simulink model "VendingMachine"  (R2025a)
settings: Solver=VariableStepAuto  StartTime=0.0  StopTime=Inf  RelTol=1e-3
settings Model: Creator=Soochan Kim  LastModifiedBy=Soochan Kim

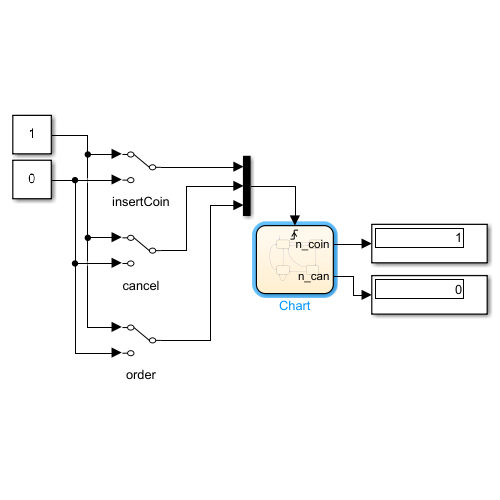
[thumbnail: Simulink's stored preview of the top-level diagram]
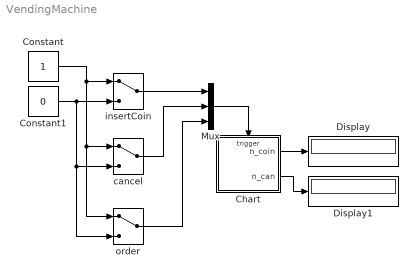
== system VendingMachine ==
  Chart : Stateflow chart  TreatAsAtomicUnit=on
  Constant : Constant
  Constant1 : Constant  Value=0
  Display : Display
  Display1 : Display
  Mux : Mux  Inputs=3
  cancel : ManualSwitch
  insertCoin : ManualSwitch
  order : ManualSwitch
  wires:
  Chart/1(n_coin) -> Display/1
  Chart/2(n_can) -> Display1/1
  Mux/1 -> Chart/Trigger
  Constant/1 -> cancel/1, order/1, insertCoin/1
  Constant1/1 -> order/2, cancel/2, insertCoin/2
  insertCoin/1 -> Mux/1
  cancel/1 -> Mux/2
  order/1 -> Mux/3

== stateflow chart VendingMachine/Chart ==
  settings: executeAtInitialization=1
  state Empty
    en:
    n_coin=0;
  state OneCoin
    entry:
    n_coin=1;
  state ThreeCoin
    en:
    n_coin=3
  state TwoCoin
    entry:
    n_coin=2;
  (default) -> Empty
  Empty -> OneCoin : insertCoin
  ThreeCoin -> Empty [order 2] : cancel
  OneCoin -> Empty [order 2] : cancel
  ThreeCoin -> Empty [order 1] : order/{n_can=1;}
  TwoCoin -> Empty [order 2] : cancel
  OneCoin -> TwoCoin [order 1] : insertCoin
  TwoCoin -> ThreeCoin [order 1] : insertCoin
  ThreeCoin -> ThreeCoin [order 3] : insertCoin
  data: n_coin output; n_can output
  events: insertCoin input RISING_EDGE_EVENT; cancel input RISING_EDGE_EVENT; order input RISING_EDGE_EVENT
